simulink model "Energy_Cost03_04_2012"  (Simulink 7.5)
settings: Solver=ode45  StartTime=0.0  StopTime=24  RelTol=1e-3
model workspace: external: MAT-File (data not in the file)
libraries: simulink x4
(part 1 of 2)
settings Model: Creator=jm3gonza  LastModifiedBy=Dr. Juan Miguel Glez
settings DebuggingCC: AlgebraicLoopMsg=none  SolverPrmCheckMsg=none  UnconnectedInputMsg=none  UnconnectedOutputMsg=none  UnconnectedLineMsg=none

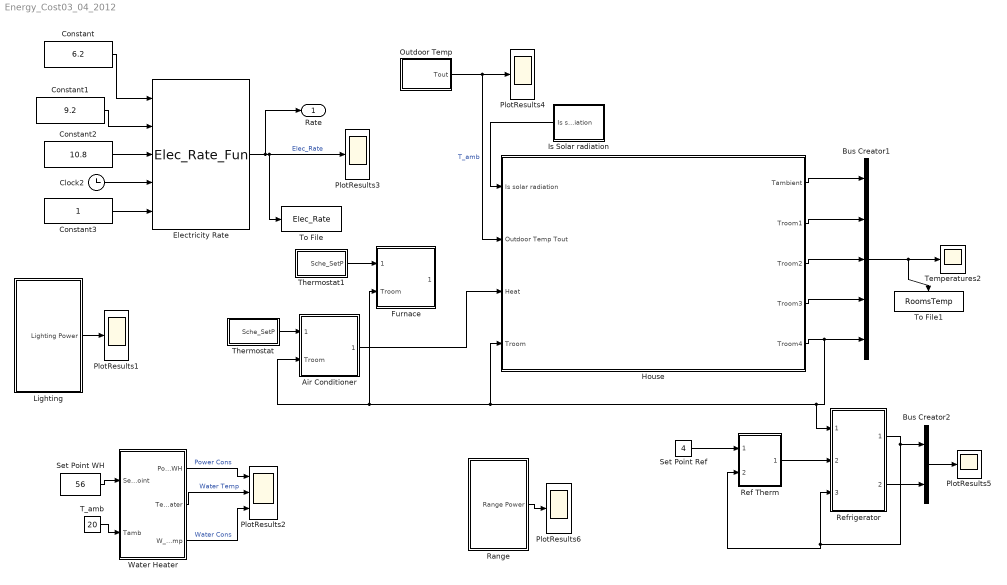
== system Energy_Cost03_04_2012 ==
  Air Conditioner : Subsystem
      mask Display:
      | % plot(-2,-2,10,12,[0 5 5 0 0], [0 0 5 5 0], [5 20 20 5], [0 0 5 5],[0 0 20 20], [5 7 7 5],...
      | %      [5 20], [1 1],[5 20], [2 2],[5 20], [3 3],[5 20], [4 4],...
      | %      [1.5 1.5], [5 7],[3 3], [5 7],[4.5 4.5], [5 7], [6 6], [5 7],[7.5 7.5], [5 7],[9 9], [5 7],...
      | %      [10.5 10.5], [5 7],[12 12], [5 7],[13.5 13.5], [5 7],[15 15], [5 7],[16.5 16.5], [5 7],[17 17], [5 7],[19 19], [5 7],...
      | %      [0 10 30 20], [7 10 10 7], [30 30 20], [10 4 0])
      | image(imread('AA.jpg'))
  Bus Creator1 : BusCreator  Inputs=5
  Bus Creator2 : BusCreator  Inputs=2
  Clock2 : Clock
      settings: Decimation=100
  Constant : Constant  Value=6.2
  Constant1 : Constant  Value=9.2
  Constant2 : Constant  Value=10.8
  Constant3 : Constant
  Electricity Rate : M-S-Function  FunctionName=Elec_Rate_Fun
      mask Display: fprintf('Elec_Rate_Fun %d',[] )
  Furnace : Subsystem
      mask Display:
      | % plot(-2,-2,10,12,[0 5 5 0 0], [0 0 5 5 0], [5 20 20 5], [0 0 5 5],[0 0 20 20], [5 7 7 5],...
      | %      [5 20], [1 1],[5 20], [2 2],[5 20], [3 3],[5 20], [4 4],...
      | %      [1.5 1.5], [5 7],[3 3], [5 7],[4.5 4.5], [5 7], [6 6], [5 7],[7.5 7.5], [5 7],[9 9], [5 7],...
      | %      [10.5 10.5], [5 7],[12 12], [5 7],[13.5 13.5], [5 7],[15 15], [5 7],[16.5 16.5], [5 7],[17 17], [5 7],[19 19], [5 7],...
      | %      [0 10 30 20], [7 10 10 7], [30 30 20], [10 4 0])
      | image(imread('Gas_Furnace.jpg'))
  House : Subsystem
      mask Display:
      | % plot([99.4454661849886;170.309218810871;170.309218810871;99.4454661849886;99.4454661849886], [212.827470386401;212.827470386401;127.790967235342;127.790967235342;212.827470386401])
      | % plot([99.4454661849886;170.309218810871], [184.481969336048;184.481969336048])
      | % plot([133.460067445412;133.460067445412], [184.481969336048;127.790967235342])
      | % plot([241.172971436754;312.036724062636;312.036724062636;241.172971436754;241.172971436754], [212.827470386401;212.827470386401;127.790967235342;127.790967235342;212.827470386401])
      | % plot([241.172971436754;312.036724062636], [184.481969336048;184.481969336048])
      | % plot([275.187572697178;275.187572697178], [184.481969336048;127.790967235342])
      | % plot([113.618216710165;42.7544640842825;368.727726163343;428.253278369084], [453.764229314402;255.34572196193;255.34572196193;453.764229314402])
      | % plot([428.253278369084;499.117030994967], [453.764229314402;382.900476688519])
      | % plot([113.618216710165;428.253278369084], [453.764229314402;453.764229314402])
      | % plot([498.86507098563;499.368991004303], [382.900476688519;382.900476688519])
      | % plot([482.109730364755;496.282480889931], [382.900476688519;382.900476688519])
      | % plot([482.109730364755;374.396826373413], [382.900476688519;275.187572697178])
      | % plot([482.109730364755;425.418728264049], [382.900476688519;439.591478789225])
      | % plot([56.927214609459;56.927214609459;354.554975638166], [255.34572196193;56.927214609459;56.927214609459])
      | % plot([354.554975638166;354.554975638166], [56.927214609459;255.34572196193])
      | % plot([354.554975638166;482.109730364755;482.109730364755], [56.927214609459;184.481969336048;382.900476688519])
      | % plot([397.073227213696;397.073227213696;439.591478789225;439.591478789225;397.073227213696], [170.309218810871;255.34572196193;297.86397353746;209.992920281366;170.309218810871])
      | % plot([397.073227213696;439.591478789225], [227.000220911577;269.518472487107])
      | % plot([419.749628053978;419.749628053978], [246.842071646824;192.985619651154])
      | % patch([0;553.20969549939;553.20969549939;0;0;0.472425017505884;0.47242501750577;552.737270481884;552.737270481885;0.472425017505884;0], [496.518693398684;496.518693398684;0;0;496.518693398684;496.046268381178;0.472425017505884;0.472425017505884;496.046268381178;496.046268381178;496.518693398684], [1;1;1])
      | image(imread('Typical-Canadian-House.jpg'))
  Is Solar radiation : Subsystem
      mask Display:
      | plot([0    0.1500    0.3000    0.4500    1.0000    1.1500    1.3000    1.4500    2.0000    2.1500    2.3000    2.4500    3.0000    3.1500    3.3000    3.4500    4.0000    4.1500    4.3000    4.4500    5.0000    5.1500    5.3000    5.4500    6.0000    6.1500    6.3000    6.4500    7.0000    7.1500    7.3000    7.4500    8.0000    8.1500    8.3000    8.4500    9.0000    9.1500    9.3000    9.4500   10.0000   10.1500   10.3000   10.4500   11.0000   11.1500   11.3000   11.4500   12.0000   12.1500   12.3000   12.4500   13.0000   13.1500   13.3000   13.4500   14.0000   14.1500   14.3000   14.4500   15.0000   15.1500   15.3000   15.4500   16.0000   16.1500   16.3000   16.4500   17.0000   17.1500   17.3000   17.4500   18.0000   18.1500   18.3000   18.4500   19.0000   19.1500   19.3000   19.4500   20.0000   20.1500   20.3000   20.4500   21.0000   21.1500   21.3000   21.4500   22.0000   22.1500   22.3000   22.4500   23.0000   23.1500   23.3000   23.4500],...
      |     [0 0 0 0 0 0 0 0 0 0 0 0 0 0 0 0 0 0 0 0 0 12.85 12.85 12.85 25.699 38.55 51.399 38.55 70.673 70.674 122.073 147.772 102.797 237.697 160.597 186.273 186.268 173.422 404.649 571.658 327.556 411.017 468.811 391.717 314.634 237.577 301.802 417.367 584.316 449.469 719.125 532.917 340.26 199.027 340.266 404.503 288.922 314.601 340.296 301.769 288.938 263.253 288.942 321.049 417.349 327.463 365.947 365.936 269.636 224.709 231.145 173.362 154.103 147.682 128.422 102.737 83.473 70.634 25.685 25.686 0 0 0 0 0 0 0 0 0 0 0 0 0 0 0 0 ])
  Lighting : Subsystem
      mask Display: image(imread('CFL_lighting.jpg'))
  Outdoor Temp : Subsystem
      mask Display:
      | plot([0    0.1500    0.3000    0.4500    1.0000    1.1500    1.3000    1.4500    2.0000    2.1500    2.3000    2.4500    3.0000    3.1500    3.3000    3.4500    4.0000    4.1500    4.3000    4.4500    5.0000    5.1500    5.3000    5.4500    6.0000    6.1500    6.3000    6.4500    7.0000    7.1500    7.3000    7.4500    8.0000    8.1500    8.3000    8.4500    9.0000    9.1500    9.3000    9.4500   10.0000   10.1500   10.3000   10.4500   11.0000   11.1500   11.3000   11.4500   12.0000   12.1500   12.3000   12.4500   13.0000   13.1500   13.3000   13.4500   14.0000   14.1500   14.3000   14.4500   15.0000   15.1500   15.3000   15.4500   16.0000   16.1500   16.3000   16.4500   17.0000   17.1500   17.3000   17.4500   18.0000   18.1500   18.3000   18.4500   19.0000   19.1500   19.3000   19.4500   20.0000   20.1500   20.3000   20.4500   21.0000   21.1500   21.3000   21.4500   22.0000   22.1500   22.3000   22.4500   23.0000   23.1500   23.3000   23.4500],...
      |     [-11.1291  -11.1588  -11.2754  -11.3348  -11.3640  -11.3349  -11.2761  -11.3644  -11.4820  -11.6877  -11.9824  -12.3084  -12.4564  -12.7586 -12.9110  -13.1851  -13.3978  -13.7036  -13.6713  -14.1054  -13.8875  -13.7327  -13.6400  -13.6400  -13.7636  -13.8879  -14.1072  -14.3577  -14.5135  -14.6391  -14.6391  -14.3243  -14.2618  -14.0769  -13.3678  -13.1847  -13.1874  -12.8845  -12.1952  -12.1968  -11.7508  -11.6376  -11.1100  -10.7030  -10.1258   -9.5609   -9.5616   -9.1089   -8.8274   -8.6038   -8.0754   -7.9926   -7.0311   -6.4872   -6.3536   -6.0586   -5.7638   -5.5768   -5.2566   -5.2045   -4.5670   -3.8272   -3.7990   -3.8776   -3.7724   -3.8777   -4.3791   -4.7245   -4.5643   -4.8546   -5.4121  -5.8135   -6.1916   -6.5106   -6.7813   -7.1642   -7.2707   -7.4860   -7.6777   -7.7616   -8.1494   -8.2612   -9.1811   -9.5460  -10.2024  -10.1740  -10.7173  -11.6519  -11.9196  -13.5221  -14.0461  -14.9577  -15.4698  -15.7285  -16.0525  -16.2152])
  PlotResults{1,3..6} (5 alike) : Scope
      PlotResults1 settings: TimeRange=24  YMin=0  YMax=130  SaveName=a1  DataFormat=Array
      PlotResults3 settings: TimeRange=25  YMin=6  YMax=11  SaveName=a  DataFormat=Array
      PlotResults4 settings: TimeRange=24  YMin=-15  YMax=25  SaveName=a3  DataFormat=Array
      PlotResults5 settings: TimeRange=24  YMin=-1  YMax=17  SaveName=a12  DataFormat=Array
      PlotResults6 settings: TimeRange=24  YMin=-1  YMax=1  SaveName=a8  DataFormat=Array
  PlotResults2 : Scope  NumInputPorts=3
      settings: TimeRange=24  YMin=0~51.5~2.5  YMax=4500~58.5~27.5  SaveName=a2  DataFormat=Array
  Range : Subsystem
      mask Display: image(imread('Stove.jpg'))
  Ref Therm : Subsystem
      mask Display: image(imread('Thermostat.jpg'))
  Refrigerator : Subsystem
      mask Display:
      | % plot(-17,-17,180,180,[0 150 150 0 0], [0 0 150 150 0],[0 80 200 150],[150 170 170 150],...
      | %     [150 200 200],[0 30 170],...
      | %     [60 60],[0 150],...
      | %     [50 50 55 55 50],[60 90 90 60 60],...
      | %     [60 60 65 65 60],[60 90 90 60 60])
      | image(imread('Refrigerator.jpg'))
  Set Point Ref : Constant  Value=4
  Set Point WH : Constant  Value=56
  T_amb : Constant  Value=20
  Temperatures2 : Scope
      settings: TimeRange=24  YMin=20  YMax=34  SaveName=a5  DataFormat=Array
  Thermostat : Subsystem
      mask Display: image(imread('Thermostat.jpg'))
  Thermostat1 : Subsystem
      mask Display: image(imread('Thermostat.jpg'))
  To File : ToFile  Filename=Elec_Rate  MatrixName=Elec_Rate
  To File1 : ToFile  Filename=RoomsTemp  MatrixName=RoomsTemp
  Water Heater : Subsystem
      mask Display: image(imread('Water_Heater.jpg'))
  Rate : Outport  InitialOutput=0
  wires:
  Constant/1 -> Electricity Rate/1
  Constant1/1 -> Electricity Rate/2
  Constant2/1 -> Electricity Rate/3
  Clock2/1 -> Electricity Rate/4
  Constant3/1 -> Electricity Rate/5
  Electricity Rate/1 -> PlotResults3/1, To File/1, Rate/1  "Elec_Rate"
  Lighting/1(Lighting Power) -> PlotResults1/1
  Set Point WH/1 -> Water Heater/1(Set point)
  T_amb/1 -> Water Heater/2(Tamb)
  Water Heater/1(Power_WH) -> PlotResults2/1  "Power Cons"
  Water Heater/2(Temp_Water) -> PlotResults2/2  "Water Temp"
  Water Heater/3(W_Consump) -> PlotResults2/3  "Water Cons"
  Outdoor Temp/1(Tout) -> PlotResults4/1, House/2(Outdoor Temp Tout)  "T_amb"
  House/5(Troom4) -> Bus Creator1/5, House/4(Troom), Air Conditioner/2(Troom), Furnace/2(Troom), Refrigerator/1(Outdoor Temp Tout)
  House/1(Tambient) -> Bus Creator1/1
  House/2(Troom1) -> Bus Creator1/2
  House/3(Troom2) -> Bus Creator1/3
  House/4(Troom3) -> Bus Creator1/4
  Bus Creator1/1 -> Temperatures2/1, To File1/1
  Air Conditioner/1(ONOFF) -> House/3(Heat)
  Is Solar radiation/1(Is solar radiation) -> House/1(Is solar radiation)
  Thermostat/1(Sche_SetP) -> Air Conditioner/1(Set point)
  Set Point Ref/1 -> Ref Therm/1(Tamb)
  Bus Creator2/1 -> PlotResults5/1
  Ref Therm/1(Ref Therm) -> Refrigerator/2(On/Off)
  Refrigerator/1(Indoor Temp) -> Bus Creator2/1, Refrigerator/3(Troom), Ref Therm/2(Tamb1)
  Range/1(Range Power) -> PlotResults6/1
  Refrigerator/2(Power_FR) -> Bus Creator2/2
  Thermostat1/1(Sche_SetP) -> Furnace/1(Set point)

== system Energy_Cost03_04_2012/Air Conditioner ==
  Set point : Inport
  Troom : Inport  Port=2
  AA or Heat : Constant
  AA_OnOff : Constant
  Cost_AA : Subsystem
      mask Display: % image(imread('Elec_stove.jpg'))
  PlotResults6 : Scope
      settings: TimeRange=24  YMin=0  YMax=1  SaveName=a9  DataFormat=Array
  Q_AA : Constant  Value=-18991793.6694
  Relay : Relay  OnSwitchValue=1.5  OffSwitchValue=-1.5  OnOutputValue=0  OffOutputValue=1
  Sum : Sum  Inputs=|+-  SampleTime=0  SaturateOnIntegerOverflow=on  InputSameDT=on  OutDataTypeStr=Inherit: Same as first input
  a : Product  Inputs=4  RndMeth=Zero
  ONOFF : Outport  InitialOutput=0
  wires:
  Set point/1 -> Sum/1
  Troom/1 -> Sum/2
  Sum/1 -> Relay/1
  Relay/1 -> a/1, PlotResults6/1
  a/1 -> ONOFF/1, Cost_AA/1(Powe_cons)
  Q_AA/1 -> a/2
  AA_OnOff/1 -> a/3
  AA or Heat/1 -> a/4

== system Energy_Cost03_04_2012/Furnace ==
  Set point : Inport
  Troom : Inport  Port=2
  AA or Heat : Constant
  AA_OnOff : Constant
  Cost_FC : Subsystem
      mask Display: % image(imread('Elec_stove.jpg'))
  PlotResults6 : Scope
      settings: TimeRange=24  YMin=-1  YMax=1  SaveName=a9  DataFormat=Array
  Q_AA : Constant  Value=-42203985.932
  Relay : Relay  OnSwitchValue=1.5  OffSwitchValue=-1.5  OnOutputValue=0  OffOutputValue=1
  Sum : Sum  Inputs=|+-  SampleTime=0  SaturateOnIntegerOverflow=on  InputSameDT=on  OutDataTypeStr=Inherit: Same as first input
  a : Product  Inputs=4  RndMeth=Zero
  ONOFF : Outport  InitialOutput=0
  wires:
  AA or Heat/1 -> a/4
  AA_OnOff/1 -> a/3
  Q_AA/1 -> a/2
  a/1 -> Cost_FC/1(Powe_cons), ONOFF/1
  Relay/1 -> PlotResults6/1, a/1
  Sum/1 -> Relay/1
  Troom/1 -> Sum/2
  Set point/1 -> Sum/1

== system Energy_Cost03_04_2012/House ==
  Is solar radiation : Inport
  Outdoor Temp Tout : Inport  Port=2
  Heat : Inport  Port=3
  Troom : Inport  Port=4
  Room_1 : Subsystem
  Room_2 : Subsystem
  Room_3 : Subsystem
  Room_4 : Subsystem
  Tambient : Outport  InitialOutput=0
  Troom1 : Outport  Port=2  InitialOutput=0
  Troom2 : Outport  Port=3  InitialOutput=0
  Troom3 : Outport  Port=4  InitialOutput=0
  Troom4 : Outport  Port=5  InitialOutput=0
  wires:
  Is solar radiation/1 -> Room_1/1(Is solar radiation), Room_2/1(Is solar radiation), Room_3/1(Is solar radiation), Room_4/1(Is solar radiation)
  Outdoor Temp Tout/1 -> Room_1/2(Outdoor Temp Tout), Room_2/2(Outdoor Temp Tout), Room_3/2(Outdoor Temp Tout), Room_4/2(Outdoor Temp Tout), Tambient/1
  Heat/1 -> Room_1/3(Q_Heat), Room_2/3(Q_Heat), Room_3/3(Q_Heat), Room_4/3(Q_Heat)  "Q_Heat"
  Troom/1 -> Room_1/4(Troom), Room_2/4(Troom), Room_3/4(Troom), Room_4/4(Troom)
  Room_1/1(Room Temp Troom) -> Troom1/1
  Room_2/1(Room Temp Troom) -> Troom2/1
  Room_3/1(Room Temp Troom) -> Troom3/1
  Room_4/1(Room Temp Troom) -> Troom4/1

== system Energy_Cost03_04_2012/Is Solar radiation ==
  Avg Outdoor Temp : Constant
  Outdoor Temp : simulink/Sources/Repeating Sequence Interpolated  SystemSampleTime=-1  OutValues=|  TimeValues=|  LookUpMeth=Interpolation-Use End Values  tsamp=-1  OutMin=[]  OutMax=[]  OutDataTypeStr=double  OutputDataTypeScalingMode=double  OutDataType=fixdt(0,8)  OutScaling=2^-10
      OutValues=|
      | [0
      | 0
      | 0
      | 0
      | 0
      | 0
      | 0
      | 0
      | 0
      | 0
      | 0
      | 0
      | 0
      | 0
      | 0
      | 0
      | 0
      | 0
      | 0
      | 0
      | 0
      | 12.85
      | 12.85
      | 12.85
      | 25.699
      | 38.55
      | 51.399
      | 38.55
      | 70.673
      | 70.674
      | 122.073
      | 147.772
      | 102.797
      | 237.697
      | 160.597
      | 186.273
      | 186.268
      | 173.422
      | 404.649
      | 571.658
      | 327.556
      | 411.017
      | 468.811
      | 391.717
      | 314.634
      | 237.577
      | 301.802
      | 417.367
      | 584.316
      | 449.469
      | 719.125
      | 532.917
      | 340.26
      | 199.027
      | 340.266
      | 404.503
      | 288.922
      | 314.601
      | 340.296
      | 301.769
      | 288.938
      | 263.253
      | 288.942
      | 321.049
      | 417.349
      | 327.463
      | 365.947
      | 365.936
      | 269.636
      | 224.709
      | 231.145
      | 173.362
      | 154.103
      | 147.682
      | 128.422
      | 102.737
      | 83.473
      | 70.634
      | 25.685
      | 25.686
      | 0
      | 0
      | 0
      | 0
      | 0
      | 0
      | 0
      | 0
      | 0
      | 0
      | 0
      | 0
      | 0
      | 0
      | 0
      | 0
      | ].'
      TimeValues=|
      | [         0
      |     0.1500
      |     0.3000
      |     0.4500
      |     1.0000
      |     1.1500
      |     1.3000
      |     1.4500
      |     2.0000
      |     2.1500
      |     2.3000
      |     2.4500
      |     3.0000
      |     3.1500
      |     3.3000
      |     3.4500
      |     4.0000
      |     4.1500
      |     4.3000
      |     4.4500
      |     5.0000
      |     5.1500
      |     5.3000
      |     5.4500
      |     6.0000
      |     6.1500
      |     6.3000
      |     6.4500
      |     7.0000
      |     7.1500
      |     7.3000
      |     7.4500
      |     8.0000
      |     8.1500
      |     8.3000
      |     8.4500
      |     9.0000
      |     9.1500
      |     9.3000
      |     9.4500
      |    10.0000
      |    10.1500
      |    10.3000
      |    10.4500
      |    11.0000
      |    11.1500
      |    11.3000
      |    11.4500
      |    12.0000
      |    12.1500
      |    12.3000
      |    12.4500
      |    13.0000
      |    13.1500
      |    13.3000
      |    13.4500
      |    14.0000
      |    14.1500
      |    14.3000
      |    14.4500
      |    15.0000
      |    15.1500
      |    15.3000
      |    15.4500
      |    16.0000
      |    16.1500
      |    16.3000
      |    16.4500
      |    17.0000
      |    17.1500
      |    17.3000
      |    17.4500
      |    18.0000
      |    18.1500
      |    18.3000
      |    18.4500
      |    19.0000
      |    19.1500
      |    19.3000
      |    19.4500
      |    20.0000
      |    20.1500
      |    20.3000
      |    20.4500
      |    21.0000
      |    21.1500
      |    21.3000
      |    21.4500
      |    22.0000
      |    22.1500
      |    22.3000
      |    22.4500
      |    23.0000
      |    23.1500
      |    23.3000
      |    23.4500].'
  Sum1 : Sum  Inputs=|++  SaturateOnIntegerOverflow=on  InputSameDT=on  OutDataTypeStr=Inherit: Same as first input
  Is solar radiation : Outport  InitialOutput=0
  wires:
  Avg Outdoor Temp/1 -> Sum1/1
  Outdoor Temp/1 -> Sum1/2
  Sum1/1 -> Is solar radiation/1

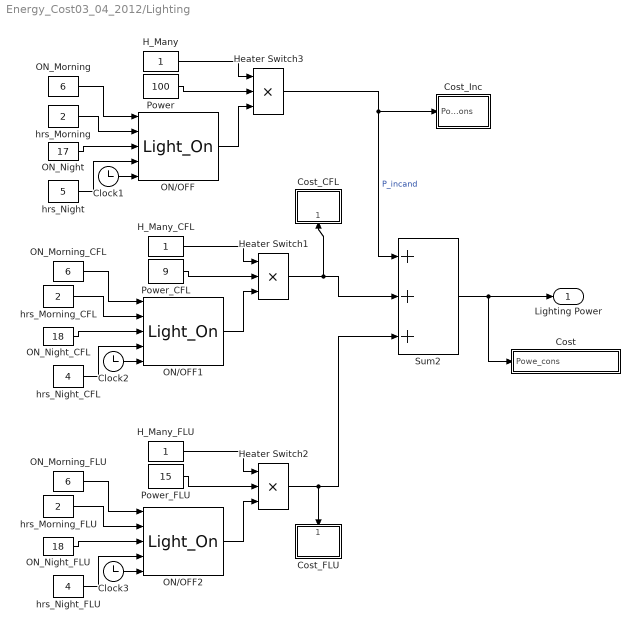
== system Energy_Cost03_04_2012/Lighting ==
  Clock1 : Clock
      settings: Decimation=100
  Clock2 : Clock
      settings: Decimation=100
  Clock3 : Clock
      settings: Decimation=100
  Cost : Subsystem
      mask Display: % image(imread('Elec_stove.jpg'))
  Cost_CFL : Subsystem
      mask Display: % image(imread('Elec_stove.jpg'))
  Cost_FLU : Subsystem
      mask Display: % image(imread('Elec_stove.jpg'))
  Cost_Inc : Subsystem
      mask Display: % image(imread('Elec_stove.jpg'))
  H_Many : Constant
  H_Many_CFL : Constant
  H_Many_FLU : Constant
  Heater Switch1 : Product  Inputs=3  RndMeth=Zero
  Heater Switch2 : Product  Inputs=3  RndMeth=Zero
  Heater Switch3 : Product  Inputs=3  RndMeth=Zero
  ON/OFF : M-S-Function  FunctionName=Light_On
      mask Display: port_label('output', 1, 'ON/OFF')
  ON/OFF1 : M-S-Function  FunctionName=Light_On
      mask Display: port_label('output', 1, 'ON/OFF')
  ON/OFF2 : M-S-Function  FunctionName=Light_On
      mask Display: port_label('output', 1, 'ON/OFF')
  ON_Morning : Constant  Value=6
  ON_Morning_CFL : Constant  Value=6
  ON_Morning_FLU : Constant  Value=6
  ON_Night : Constant  Value=17
  ON_Night_CFL : Constant  Value=18
  ON_Night_FLU : Constant  Value=18
  Power : Constant  Value=100
  Power_CFL : Constant  Value=9
  Power_FLU : Constant  Value=15
  Sum2 : Sum  Inputs=+++  SaturateOnIntegerOverflow=on  InputSameDT=on  OutDataTypeStr=Inherit: Same as first input
  hrs_Morning : Constant  Value=2
  hrs_Morning_CFL : Constant  Value=2
  hrs_Morning_FLU : Constant  Value=2
  hrs_Night : Constant  Value=5
  hrs_Night_CFL : Constant  Value=4
  hrs_Night_FLU : Constant  Value=4
  Lighting Power : Outport  InitialOutput=0
  wires:
  H_Many/1 -> Heater Switch3/1
  Power/1 -> Heater Switch3/2
  Heater Switch3/1 -> Cost_Inc/1(Powe_cons), Sum2/1  "P_incand"
  ON/OFF/1 -> Heater Switch3/3
  Clock1/1 -> ON/OFF/5
  hrs_Morning/1 -> ON/OFF/2
  ON_Night/1 -> ON/OFF/3
  hrs_Night/1 -> ON/OFF/4
  ON_Morning/1 -> ON/OFF/1
  H_Many_CFL/1 -> Heater Switch1/1
  Power_CFL/1 -> Heater Switch1/2
  ON/OFF1/1 -> Heater Switch1/3
  Clock2/1 -> ON/OFF1/5
  hrs_Morning_CFL/1 -> ON/OFF1/2
  ON_Night_CFL/1 -> ON/OFF1/3
  hrs_Night_CFL/1 -> ON/OFF1/4
  ON_Morning_CFL/1 -> ON/OFF1/1
  H_Many_FLU/1 -> Heater Switch2/1
  Power_FLU/1 -> Heater Switch2/2
  ON/OFF2/1 -> Heater Switch2/3
  Clock3/1 -> ON/OFF2/5
  hrs_Morning_FLU/1 -> ON/OFF2/2
  ON_Night_FLU/1 -> ON/OFF2/3
  hrs_Night_FLU/1 -> ON/OFF2/4
  ON_Morning_FLU/1 -> ON/OFF2/1
  Heater Switch1/1 -> Sum2/2, Cost_CFL/1(Powe_cons)
  Heater Switch2/1 -> Sum2/3, Cost_FLU/1(Powe_cons)
  Sum2/1 -> Lighting Power/1, Cost/1(Powe_cons)

== system Energy_Cost03_04_2012/Outdoor Temp ==
  Heater Switch1 : Product  RndMeth=Zero
  Heater Switch2 : Product  RndMeth=Zero
  Sum2 : Sum  SaturateOnIntegerOverflow=on  InputSameDT=on  OutDataTypeStr=Inherit: Same as first input
  Summer : simulink/Sources/Repeating Sequence Interpolated  SystemSampleTime=-1  OutValues=|  TimeValues=|  LookUpMeth=Interpolation-Use End Values  tsamp=-1  OutMin=[]  OutMax=[]  OutDataTypeStr=double  OutputDataTypeScalingMode=double  OutDataType=fixdt(0,8)  OutScaling=2^-10
      OutValues=|
      | [   23.8160
      |    23.7130
      |    23.4480
      |    23.2590
      |    23.1710
      |    23.1330
      |    22.9330
      |    22.8600
      |    22.7100
      |    22.6330
      |    22.4980
      |    22.3130
      |    22.2390
      |    22.1040
      |    21.9830
      |    21.7030
      |    21.5360
      |    21.4650
      |    21.8150
      |    22.1730
      |    22.3830
      |    22.6540
      |    22.7390
      |    22.9630
      |    23.3760
      |    23.9600
      |    24.3460
      |    24.7420
      |    24.9870
      |    25.3280
      |    25.6220
      |    26.4600
      |    26.8940
      |    27.7100
      |    27.9620
      |    28.1630
      |    28.4950
      |    29.0620
      |    29.0190
      |    29.0170
      |    29.2500
      |    29.6940
      |    29.8860
      |    29.9560
      |    30.0730
      |    30.6760
      |    30.8120
      |    30.9150
      |    31.2920
      |    30.8100
      |    31.3250
      |    31.3570
      |    31.6710
      |    32.3710
      |    31.6010
      |    32.0310
      |    32.1090
      |    32.3180
      |    32.3980
      |    31.7870
      |    31.6290
      |    33.0060
      |    33.0040
      |    32.8570
      |    32.9240
      |    32.6620
      |    33.1210
      |    32.6940
      |    32.3640
      |    32.0100
      |    31.5350
      |    32.0310
      |    31.0020
      |    30.4620
      |    30.0880
      |    29.8870
      |    29.5410
      |    29.3690
      |    29.1040
      |    28.6390
      |    28.1200
      |    26.7970
      |    26.0180
      |    25.6170
      |    26.9460
      |    27.3140
      |    27.1220
      |    26.8170
      |    26.5690
      |    26.4040
      |    26.2680
      |    26.1190
      |    25.7690
      |    25.4730
      |    25.2080
      |    24.9570].'
      TimeValues=|
      | [         0
      |     0.1500
      |     0.3000
      |     0.4500
      |     1.0000
      |     1.1500
      |     1.3000
      |     1.4500
      |     2.0000
      |     2.1500
      |     2.3000
      |     2.4500
      |     3.0000
      |     3.1500
      |     3.3000
      |     3.4500
      |     4.0000
      |     4.1500
      |     4.3000
      |     4.4500
      |     5.0000
      |     5.1500
      |     5.3000
      |     5.4500
      |     6.0000
      |     6.1500
      |     6.3000
      |     6.4500
      |     7.0000
      |     7.1500
      |     7.3000
      |     7.4500
      |     8.0000
      |     8.1500
      |     8.3000
      |     8.4500
      |     9.0000
      |     9.1500
      |     9.3000
      |     9.4500
      |    10.0000
      |    10.1500
      |    10.3000
      |    10.4500
      |    11.0000
      |    11.1500
      |    11.3000
      |    11.4500
      |    12.0000
      |    12.1500
      |    12.3000
      |    12.4500
      |    13.0000
      |    13.1500
      |    13.3000
      |    13.4500
      |    14.0000
      |    14.1500
      |    14.3000
      |    14.4500
      |    15.0000
      |    15.1500
      |    15.3000
      |    15.4500
      |    16.0000
      |    16.1500
      |    16.3000
      |    16.4500
      |    17.0000
      |    17.1500
      |    17.3000
      |    17.4500
      |    18.0000
      |    18.1500
      |    18.3000
      |    18.4500
      |    19.0000
      |    19.1500
      |    19.3000
      |    19.4500
      |    20.0000
      |    20.1500
      |    20.3000
      |    20.4500
      |    21.0000
      |    21.1500
      |    21.3000
      |    21.4500
      |    22.0000
      |    22.1500
      |    22.3000
      |    22.4500
      |    23.0000
      |    23.1500
      |    23.3000
      |    23.4500].'
  Temp_aux : Constant  SampleTime=0
  Temp_aux1 : Constant  Value=0  SampleTime=0
  Winter : simulink/Sources/Repeating Sequence Interpolated  SystemSampleTime=-1  OutValues=|  TimeValues=|  LookUpMeth=Interpolation-Use End Values  tsamp=-1  OutMin=[]  OutMax=[]  OutDataTypeStr=double  OutputDataTypeScalingMode=double  OutDataType=fixdt(0,8)  OutScaling=2^-10
      OutValues=|
      | [  -11.1291
      |   -11.1588
      |   -11.2754
      |   -11.3348
      |   -11.3640
      |   -11.3349
      |   -11.2761
      |   -11.3644
      |   -11.4820
      |   -11.6877
      |   -11.9824
      |   -12.3084
      |   -12.4564
      |   -12.7586
      |   -12.9110
      |   -13.1851
      |   -13.3978
      |   -13.7036
      |   -13.6713
      |   -14.1054
      |   -13.8875
      |   -13.7327
      |   -13.6400
      |   -13.6400
      |   -13.7636
      |   -13.8879
      |   -14.1072
      |   -14.3577
      |   -14.5135
      |   -14.6391
      |   -14.6391
      |   -14.3243
      |   -14.2618
      |   -14.0769
      |   -13.3678
      |   -13.1847
      |   -13.1874
      |   -12.8845
      |   -12.1952
      |   -12.1968
      |   -11.7508
      |   -11.6376
      |   -11.1100
      |   -10.7030
      |   -10.1258
      |    -9.5609
      |    -9.5616
      |    -9.1089
      |    -8.8274
      |    -8.6038
      |    -8.0754
      |    -7.9926
      |    -7.0311
      |    -6.4872
      |    -6.3536
      |    -6.0586
      |    -5.7638
      |    -5.5768
      |    -5.2566
      |    -5.2045
      |    -4.5670
      |    -3.8272
      |    -3.7990
      |    -3.8776
      |    -3.7724
      |    -3.8777
      |    -4.3791
      |    -4.7245
      |    -4.5643
      |    -4.8546
      |    -5.4121
      |    -5.8135
      |    -6.1916
      |    -6.5106
      |    -6.7813
      |    -7.1642
      |    -7.2707
      |    -7.4860
      |    -7.6777
      |    -7.7616
      |    -8.1494
      |    -8.2612
      |    -9.1811
      |    -9.5460
      |   -10.2024
      |   -10.1740
      |   -10.7173
      |   -11.6519
      |   -11.9196
      |   -13.5221
      |   -14.0461
      |   -14.9577
      |   -15.4698
      |   -15.7285
      |   -16.0525
      |   -16.2152
      |   -16.2152
      |   -16.52].'
      TimeValues=|
      | [         0
      |     0.1500
      |     0.3000
      |     0.4500
      |     1.0000
      |     1.1500
      |     1.3000
      |     1.4500
      |     2.0000
      |     2.1500
      |     2.3000
      |     2.4500
      |     3.0000
      |     3.1500
      |     3.3000
      |     3.4500
      |     4.0000
      |     4.1500
      |     4.3000
      |     4.4500
      |     5.0000
      |     5.1500
      |     5.3000
      |     5.4500
      |     6.0000
      |     6.1500
      |     6.3000
      |     6.4500
      |     7.0000
      |     7.1500
      |     7.3000
      |     7.4500
      |     8.0000
      |     8.1500
      |     8.3000
      |     8.4500
      |     9.0000
      |     9.1500
      |     9.3000
      |     9.4500
      |    10.0000
      |    10.1500
      |    10.3000
      |    10.4500
      |    11.0000
      |    11.1500
      |    11.3000
      |    11.4500
      |    12.0000
      |    12.1500
      |    12.3000
      |    12.4500
      |    13.0000
      |    13.1500
      |    13.3000
      |    13.4500
      |    14.0000
      |    14.1500
      |    14.3000
      |    14.4500
      |    15.0000
      |    15.1500
      |    15.3000
      |    15.4500
      |    16.0000
      |    16.1500
      |    16.3000
      |    16.4500
      |    17.0000
      |    17.1500
      |    17.3000
      |    17.4500
      |    18.0000
      |    18.1500
      |    18.3000
      |    18.4500
      |    19.0000
      |    19.1500
      |    19.3000
      |    19.4500
      |    20.0000
      |    20.1500
      |    20.3000
      |    20.4500
      |    21.0000
      |    21.1500
      |    21.3000
      |    21.4500
      |    22.0000
      |    22.1500
      |    22.3000
      |    22.4500
      |    23.0000
      |    23.1500
      |    23.3000
      |    23.4500
      |    23.900  
      |    24.000].'
  Tout : Outport  InitialOutput=0
  wires:
  Heater Switch1/1 -> Sum2/1  "Toutdoors"
  Temp_aux/1 -> Heater Switch1/1
  Summer/1 -> Heater Switch1/2
  Heater Switch2/1 -> Sum2/2  "Toutdoors"
  Temp_aux1/1 -> Heater Switch2/1
  Winter/1 -> Heater Switch2/2
  Sum2/1 -> Tout/1

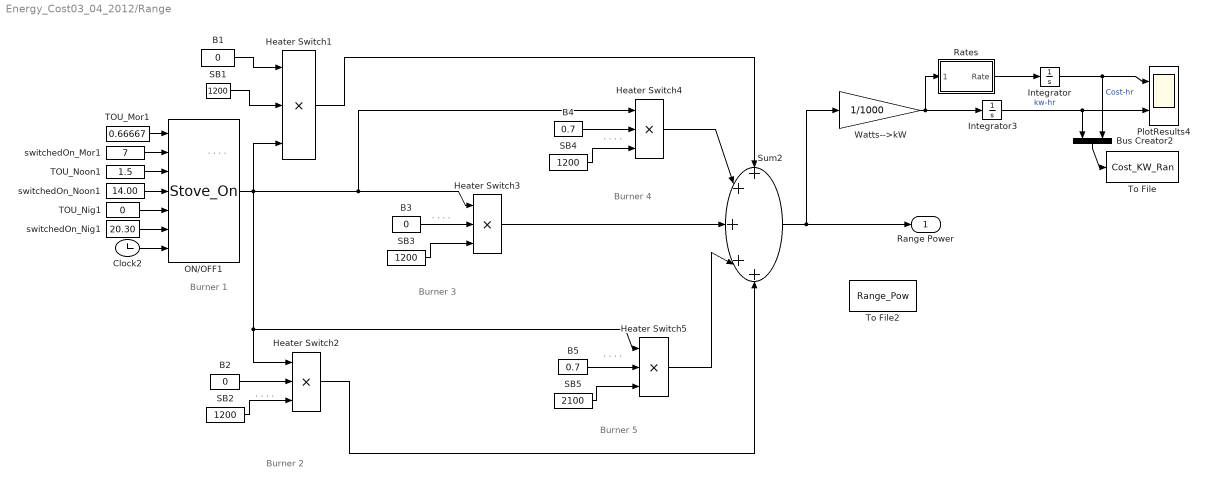
== system Energy_Cost03_04_2012/Range ==
  note: Burner 1
  note: Burner 2
  note: Burner 3
  note: Burner 4
  note: Burner 5
  note: .                                                                                     .
      |
      |
      |
      |
      |
      |
      |
      |
      |
      |
      |
      |
      |
      |
      |
      |
      |
      |
      | .                                                                                     .
  note: .                                             .
      |
      |
      |
      |
      |
      |
      | .                                             .
  note: .                                             .
      |
      |
      |
      |
      |
      |
      | .                                             .
  note: .                                             .
      |
      |
      |
      |
      |
      |
      | .                                             .
  note: .                                             .
      |
      |
      |
      |
      |
      |
      | .                                             .
  B1 : Constant  Value=0
  B2 : Constant  Value=0
  B3 : Constant  Value=0
  B4 : Constant  Value=0.7
  B5 : Constant  Value=0.7
  Bus Creator2 : BusCreator  Inputs=2
  Clock2 : Clock
      settings: Decimation=100
  Heater Switch{1..5} (5 alike) : Product  Inputs=3  RndMeth=Zero
  Integrator : Integrator
  Integrator3 : Integrator
  ON/OFF1 : M-S-Function  FunctionName=Stove_On
      mask Display: port_label('output', 1, 'ON/OFF')
  PlotResults4 : Scope  NumInputPorts=2
      settings: TimeRange=24  YMin=0~0  YMax=37.5~3.75  SaveName=a17  DataFormat=Array
  Rates : Subsystem
      mask Display: % image(imread('Elec_stove.jpg'))
  SB{1..4} (4 alike) : Constant  Value=1200
  SB5 : Constant  Value=2100
  Sum2 : Sum  Inputs=+++++  SaturateOnIntegerOverflow=on  InputSameDT=on  OutDataTypeStr=Inherit: Same as first input
  TOU_Mor1 : Constant  Value=0.66667
  TOU_Nig1 : Constant  Value=0
  TOU_Noon1 : Constant  Value=1.5
  To File : ToFile  Filename=Cost_KW_Ran  MatrixName=Cost_KW
  To File2 : ToFile  Filename=Range_Pow  MatrixName=Range_Pow
  Watts-->kW : Gain  Gain=1/1000  SaturateOnIntegerOverflow=on  OutDataTypeStr=Inherit: Same as input  ParamDataTypeStr=Inherit: Same as input
  switchedOn_Mor1 : Constant  Value=7
  switchedOn_Nig1 : Constant  Value=20.30
  switchedOn_Noon1 : Constant  Value=14.00
  Range Power : Outport  InitialOutput=0
  wires:
  Rates/1(Rate) -> Integrator/1
  Watts-->kW/1 -> Integrator3/1, Rates/1(Powe_cons)
  Integrator3/1 -> PlotResults4/2, Bus Creator2/1  "kw-hr"
  Bus Creator2/1 -> To File/1
  Integrator/1 -> PlotResults4/1, Bus Creator2/2  "Cost-hr"
  TOU_Mor1/1 -> ON/OFF1/1
  switchedOn_Mor1/1 -> ON/OFF1/2
  Clock2/1 -> ON/OFF1/7
  TOU_Noon1/1 -> ON/OFF1/3
  switchedOn_Noon1/1 -> ON/OFF1/4
  TOU_Nig1/1 -> ON/OFF1/5
  switchedOn_Nig1/1 -> ON/OFF1/6
  B1/1 -> Heater Switch1/1
  SB1/1 -> Heater Switch1/2
  ON/OFF1/1 -> Heater Switch1/3, Heater Switch3/1, Heater Switch4/1, Heater Switch2/1, Heater Switch5/1
  SB2/1 -> Heater Switch2/3
  B2/1 -> Heater Switch2/2
  SB3/1 -> Heater Switch3/3
  B3/1 -> Heater Switch3/2
  SB4/1 -> Heater Switch4/3
  B4/1 -> Heater Switch4/2
  SB5/1 -> Heater Switch5/3
  B5/1 -> Heater Switch5/2
  Heater Switch1/1 -> Sum2/1
  Heater Switch4/1 -> Sum2/2
  Heater Switch3/1 -> Sum2/3
  Heater Switch5/1 -> Sum2/4
  Heater Switch2/1 -> Sum2/5
  Sum2/1 -> Range Power/1, Watts-->kW/1

== system Energy_Cost03_04_2012/Ref Therm ==
  Tamb : Inport
  Tamb1 : Inport  Port=2
  Sum3 : Sum  Inputs=|+-  SampleTime=0  SaturateOnIntegerOverflow=on  InputSameDT=on  OutDataTypeStr=Inherit: Same as first input
  Thermostat1 : Relay  OnSwitchValue=1.5  OffSwitchValue=-1.5  OnOutputValue=0  OffOutputValue=1  ZeroCross=off  SampleTime=0.14
  Ref Therm : Outport  InitialOutput=0
  wires:
  Sum3/1 -> Thermostat1/1
  Thermostat1/1 -> Ref Therm/1
  Tamb/1 -> Sum3/1
  Tamb1/1 -> Sum3/2

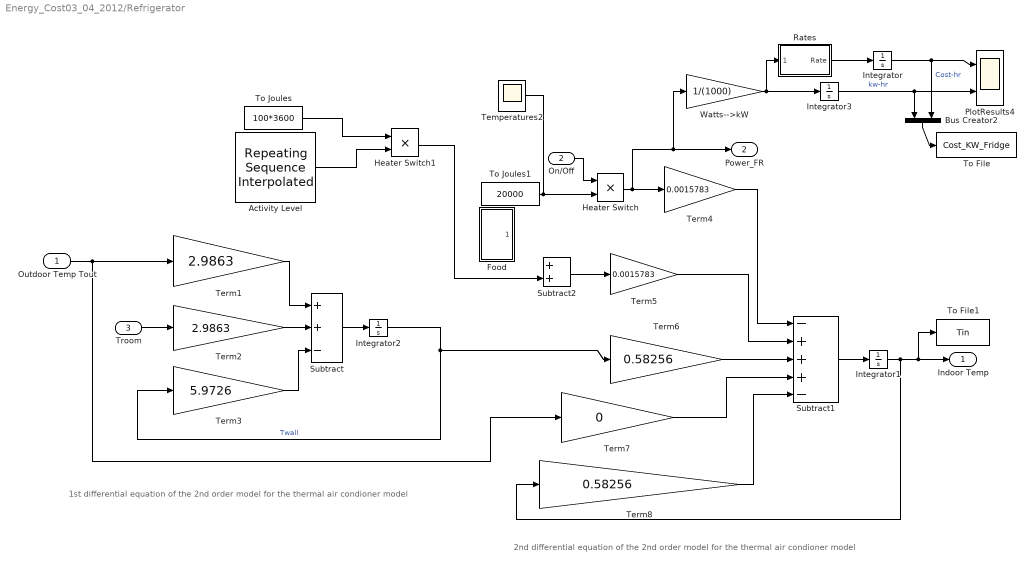
== system Energy_Cost03_04_2012/Refrigerator ==
  note: 1st differential equation of the 2nd order
      | model for the thermal air condioner model
  note: 2nd differential equation of the 2nd order
      | model for the thermal air condioner model
  Outdoor Temp Tout : Inport
  On/Off : Inport  Port=2
  Troom : Inport  Port=3
  Activity Level : simulink/Sources/Repeating Sequence Interpolated  SystemSampleTime=-1  OutValues=|  TimeValues=|  LookUpMeth=Interpolation-Use End Values  tsamp=0.1  OutMin=[]  OutMax=[]  OutDataTypeStr=double  OutputDataTypeScalingMode=double  OutDataType=fixdt(0,8)  OutScaling=2^-10
      OutValues=|
      | [         0
      |          0
      |     0.0700
      |     0.0700
      |          0
      |          0
      |     0.1000
      |     0.1000
      |          0
      |          0
      |     0.1300
      |     0.1300
      |          0
      |          0
      |     0.0300
      |     0.0300
      |          0
      |          0
      |          0
      |     0.0700
      |     0.0700
      |          0
      |          0
      |     0.1700
      |     0.1700
      |          0
      |          0
      |     0.2300
      |     0.2300
      |          0
      |          0
      |     0.1300
      |     0.1300
      |          0
      |          0
      |     0.0700
      |     0.0700
      |          0
      |          0].'
      TimeValues=|
      | [                   0
      |    9.299899999999999
      |    9.300000000000001
      |    9.303990000000001
      |    9.304000000000000
      |    9.749000000000001
      |    9.750000000000000
      |    9.755000000000001
      |    9.756000000000000
      |    9.999000000000001
      |   10.000000000000000
      |   10.006700000000000
      |   10.006800000000000
      |   10.149900000000001
      |   10.150000000000000
      |   10.151600000000000
      |   10.151700000000000
      |   10.300100000000000
      |   13.299899999999999
      |   13.300000000000001
      |   13.303300000000000
      |   13.303400000000000
      |   13.449900000000000
      |   13.449999999999999
      |   13.458399999999999
      |   13.458500000000001
      |   13.999900000000000
      |   14.000000000000000
      |   14.011690000000000
      |   14.011699999999999
      |   14.149900000000001
      |   14.150000000000000
      |   14.156700000000001
      |   14.156800000000000
      |   14.299899999999999
      |   14.300000000000001
      |   14.303300000000000
      |   14.303400000000000
      |   24.000000000000000].'
  Bus Creator2 : BusCreator  Inputs=2
  Food : Subsystem
  Heater Switch : Product  RndMeth=Zero
  Heater Switch1 : Product  RndMeth=Zero
  Integrator : Integrator
  Integrator1 : Integrator  InitialCondition=4
  Integrator2 : Integrator  InitialCondition=21
  Integrator3 : Integrator
  PlotResults4 : Scope  NumInputPorts=2
      settings: TimeRange=24  YMin=32.5~5.5  YMax=70~11.25  SaveName=a7  DataFormat=Array
  Rates : Subsystem
      mask Display: % image(imread('Elec_stove.jpg'))
  Subtract : Sum  Inputs=++-
  Subtract1 : Sum  Inputs=-+++-
  Subtract2 : Sum
  Temperatures2 : Scope
      settings: TimeRange=24  YMin=0  YMax=21000  SaveName=a13  DataFormat=Array
  Term1 : Gain  Gain=2.9863
  Term2 : Gain  Gain=2.9863
  Term3 : Gain  Gain=5.9726
  Term4 : Gain  Gain=0.0015783
  Term5 : Gain  Gain=0.0015783
  Term6 : Gain  Gain=0.58256
  Term7 : Gain  Gain=0
  Term8 : Gain  Gain=0.58256
  To File : ToFile  Filename=Cost_KW_Fridge  MatrixName=Cost_KW_Fridge
  To File1 : ToFile  Filename=Tin  MatrixName=Tin
  To Joules : Constant  Value=100*3600
  To Joules1 : Constant  Value=20000
  Watts-->kW : Gain  Gain=1/(1000)  SaturateOnIntegerOverflow=on  OutDataTypeStr=Inherit: Same as input  ParamDataTypeStr=Inherit: Same as input
  Indoor Temp : Outport  InitialOutput=0
  Power_FR : Outport  Port=2  InitialOutput=0
  wires:
  Term3/1 -> Subtract/3
  Subtract/1 -> Integrator2/1
  Integrator2/1 -> Term3/1, Term6/1  "Twall"
  Integrator1/1 -> Indoor Temp/1, To File1/1, Term8/1
  Subtract1/1 -> Integrator1/1
  Outdoor Temp Tout/1 -> Term7/1, Term1/1
  Troom/1 -> Term2/1
  Term5/1 -> Subtract1/2
  Term6/1 -> Subtract1/3
  Term7/1 -> Subtract1/4
  Term8/1 -> Subtract1/5
  Activity Level/1 -> Heater Switch1/2
  To Joules/1 -> Heater Switch1/1
  Heater Switch1/1 -> Subtract2/2
  On/Off/1 -> Heater Switch/1
  Subtract2/1 -> Term5/1
  Term1/1 -> Subtract/1
  Term2/1 -> Subtract/2
  To Joules1/1 -> Temperatures2/1, Heater Switch/2
  Heater Switch/1 -> Term4/1, Power_FR/1, Watts-->kW/1
  Term4/1 -> Subtract1/1
  Rates/1(Rate) -> Integrator/1
  Watts-->kW/1 -> Integrator3/1, Rates/1(Powe_cons)
  Integrator3/1 -> PlotResults4/2, Bus Creator2/1  "kw-hr"
  Bus Creator2/1 -> To File/1
  Integrator/1 -> PlotResults4/1, Bus Creator2/2  "Cost-hr"

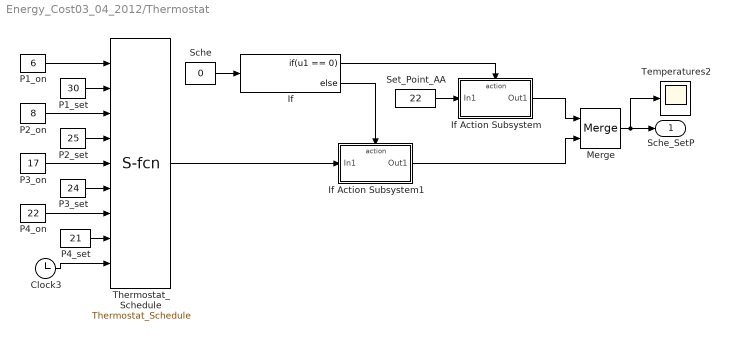
== system Energy_Cost03_04_2012/Thermostat ==
  Clock3 : Clock
      settings: Decimation=100
  If : If  IfExpression=u1 == 0
  If Action Subsystem : Subsystem  TreatAsAtomicUnit=on
  If Action Subsystem1 : Subsystem  TreatAsAtomicUnit=on
  Merge : Merge
  P1_on : Constant  Value=6
  P1_set : Constant  Value=30
  P2_on : Constant  Value=8
  P2_set : Constant  Value=25
  P3_on : Constant  Value=17
  P3_set : Constant  Value=24
  P4_on : Constant  Value=22
  P4_set : Constant  Value=21
  Sche : Constant  Value=0
  Set_Point_AA : Constant  Value=22
  Temperatures2 : Scope
      settings: TimeRange=24  YMin=21  YMax=21  SaveName=a4  DataFormat=Array
  Thermostat_Schedule : M-S-Function  FunctionName=Thermostat_Schedule
      mask Display: port_label('output', 1, 'ON/OFF')
  Sche_SetP : Outport  InitialOutput=0
  wires:
  P1_on/1 -> Thermostat_Schedule/1
  P1_set/1 -> Thermostat_Schedule/2
  P2_on/1 -> Thermostat_Schedule/3
  P2_set/1 -> Thermostat_Schedule/4
  P3_on/1 -> Thermostat_Schedule/5
  P3_set/1 -> Thermostat_Schedule/6
  P4_on/1 -> Thermostat_Schedule/7
  P4_set/1 -> Thermostat_Schedule/8
  Clock3/1 -> Thermostat_Schedule/9
  Sche/1 -> If/1
  If/1 -> If Action Subsystem/Action
  Set_Point_AA/1 -> If Action Subsystem/1(In1)
  If/2 -> If Action Subsystem1/Action
  Merge/1 -> Sche_SetP/1, Temperatures2/1
  Thermostat_Schedule/1 -> If Action Subsystem1/1(In1)
  If Action Subsystem1/1(Out1) -> Merge/2
  If Action Subsystem/1(Out1) -> Merge/1

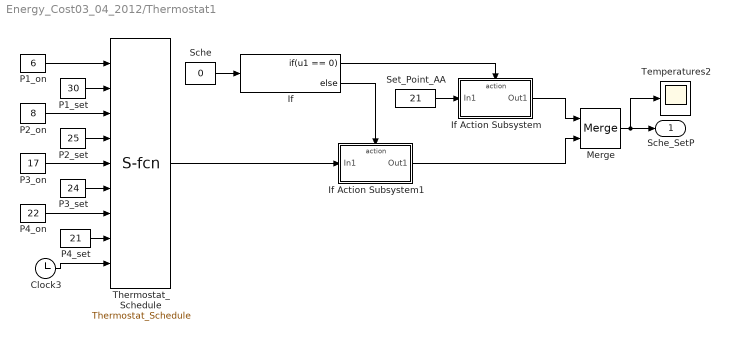
== system Energy_Cost03_04_2012/Thermostat1 ==
  Clock3 : Clock
      settings: Decimation=100
  If : If  IfExpression=u1 == 0
  If Action Subsystem : Subsystem  TreatAsAtomicUnit=on
  If Action Subsystem1 : Subsystem  TreatAsAtomicUnit=on
  Merge : Merge
  P1_on : Constant  Value=6
  P1_set : Constant  Value=30
  P2_on : Constant  Value=8
  P2_set : Constant  Value=25
  P3_on : Constant  Value=17
  P3_set : Constant  Value=24
  P4_on : Constant  Value=22
  P4_set : Constant  Value=21
  Sche : Constant  Value=0
  Set_Point_AA : Constant  Value=21
  Temperatures2 : Scope
      settings: TimeRange=24  YMin=21  YMax=21  SaveName=a4  DataFormat=Array
  Thermostat_Schedule : M-S-Function  FunctionName=Thermostat_Schedule
      mask Display: port_label('output', 1, 'ON/OFF')
  Sche_SetP : Outport  InitialOutput=0
  wires:
  P1_on/1 -> Thermostat_Schedule/1
  P1_set/1 -> Thermostat_Schedule/2
  P2_on/1 -> Thermostat_Schedule/3
  P2_set/1 -> Thermostat_Schedule/4
  P3_on/1 -> Thermostat_Schedule/5
  P3_set/1 -> Thermostat_Schedule/6
  P4_on/1 -> Thermostat_Schedule/7
  P4_set/1 -> Thermostat_Schedule/8
  Clock3/1 -> Thermostat_Schedule/9
  Sche/1 -> If/1
  If/1 -> If Action Subsystem/Action
  Set_Point_AA/1 -> If Action Subsystem/1(In1)
  If/2 -> If Action Subsystem1/Action
  Merge/1 -> Sche_SetP/1, Temperatures2/1
  Thermostat_Schedule/1 -> If Action Subsystem1/1(In1)
  If Action Subsystem1/1(Out1) -> Merge/2
  If Action Subsystem/1(Out1) -> Merge/1

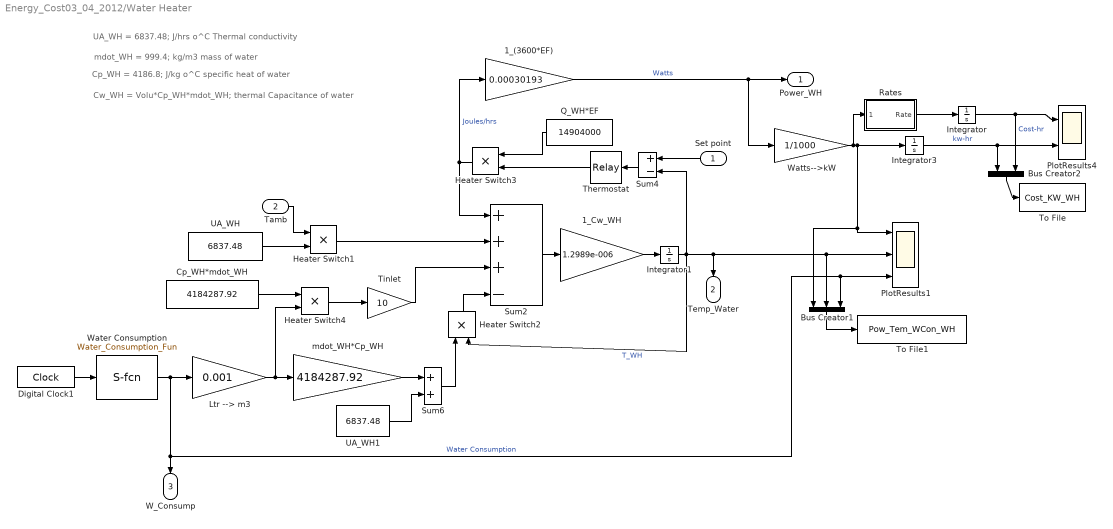
== system Energy_Cost03_04_2012/Water Heater ==
  note: UA_WH = 6837.48; J/hrs o^C Thermal conductivity
  note: mdot_WH = 999.4; kg/m3 mass of water
  note: Cp_WH = 4186.8; J/kg o^C specific heat of water
  note: Cw_WH = Volu*Cp_WH*mdot_WH; thermal Capacitance of water
  Set point : Inport
  Tamb : Inport  Port=2
  1_(3600*EF) : Gain  Gain=0.00030193  SaturateOnIntegerOverflow=on  OutDataTypeStr=Inherit: Same as input  ParamDataTypeStr=Inherit: Same as input
  1_Cw_WH : Gain  Gain=1.2989e-006  SaturateOnIntegerOverflow=on  OutDataTypeStr=Inherit: Same as input  ParamDataTypeStr=Inherit: Same as input
  Bus Creator1 : BusCreator  Inputs=3
  Bus Creator2 : BusCreator  Inputs=2
  Cp_WH*mdot_WH : Constant  Value=4184287.92
  Digital Clock1 : DigitalClock
  Heater Switch{1..4} (4 alike) : Product  RndMeth=Zero
  Integrator : Integrator
  Integrator1 : Integrator  InitialCondition=55
  Integrator3 : Integrator
  Ltr --> m3 : Gain  Gain=0.001
  PlotResults1 : Scope  NumInputPorts=3
      settings: TimeRange=24  YMin=0~42~2.5  YMax=4.5~55~27.5  SaveName=a11  DataFormat=Array
  PlotResults4 : Scope  NumInputPorts=2
      settings: TimeRange=24  YMin=47.5~13.75  YMax=67.5~18.5  SaveName=a14  DataFormat=Array
  Q_WH*EF : Constant  Value=14904000  VectorParams1D=off
  Rates : Subsystem
      mask Display: % image(imread('Elec_stove.jpg'))
  Sum2 : Sum  Inputs=+++-  SaturateOnIntegerOverflow=on  InputSameDT=on  OutDataTypeStr=Inherit: Same as first input
  Sum4 : Sum  Inputs=+-  SaturateOnIntegerOverflow=on  InputSameDT=on  OutDataTypeStr=Inherit: Same as first input
  Sum6 : Sum  SaturateOnIntegerOverflow=on  InputSameDT=on  OutDataTypeStr=Inherit: Same as first input
  Thermostat : Relay  OnSwitchValue=3  OffSwitchValue=-3
  Tinlet : Gain  Gain=10  SaturateOnIntegerOverflow=on  OutDataTypeStr=Inherit: Same as input  ParamDataTypeStr=Inherit: Same as input
  To File : ToFile  Filename=Cost_KW_WH  MatrixName=Cost_KW_WH
  To File1 : ToFile  Filename=Pow_Tem_WCon_WH  MatrixName=Pow_Tem_WCon_WH
  UA_WH : Constant  Value=6837.48
  UA_WH1 : Constant  Value=6837.48
  Water Consumption : M-S-Function  FunctionName=Water_Consumption_Fun
      mask Display: image(imread('Water_Cons.jpg'))
  Watts-->kW : Gain  Gain=1/1000  SaturateOnIntegerOverflow=on  OutDataTypeStr=Inherit: Same as input  ParamDataTypeStr=Inherit: Same as input
  mdot_WH*Cp_WH : Gain  Gain=4184287.92  SaturateOnIntegerOverflow=on  OutDataTypeStr=Inherit: Same as input  ParamDataTypeStr=Inherit: Same as input
  Power_WH : Outport  InitialOutput=0
  Temp_Water : Outport  Port=2  InitialOutput=0
  W_Consump : Outport  Port=3  InitialOutput=0
  wires:
  Sum2/1 -> 1_Cw_WH/1
  1_Cw_WH/1 -> Integrator1/1
  Digital Clock1/1 -> Water Consumption/1
  Water Consumption/1 -> Ltr --> m3/1, W_Consump/1, PlotResults1/3, Bus Creator1/3  "Water Consumption"
  UA_WH/1 -> Heater Switch1/2
  Ltr --> m3/1 -> mdot_WH*Cp_WH/1, Heater Switch4/2
  mdot_WH*Cp_WH/1 -> Sum6/1
  UA_WH1/1 -> Sum6/2
  Sum6/1 -> Heater Switch2/1
  Integrator1/1 -> Heater Switch2/2, Sum4/2, Temp_Water/1, PlotResults1/2, Bus Creator1/2  "T_WH"
  Heater Switch2/1 -> Sum2/4
  Cp_WH*mdot_WH/1 -> Heater Switch4/1
  Heater Switch4/1 -> Tinlet/1
  Tinlet/1 -> Sum2/3
  Heater Switch1/1 -> Sum2/2
  Set point/1 -> Sum4/1
  Sum4/1 -> Thermostat/1
  Q_WH*EF/1 -> Heater Switch3/1
  Heater Switch3/1 -> Sum2/1, 1_(3600*EF)/1  "Joules/hrs"
  1_(3600*EF)/1 -> Power_WH/1, Watts-->kW/1  "Watts"
  Thermostat/1 -> Heater Switch3/2
  Tamb/1 -> Heater Switch1/1
  Rates/1(Rate) -> Integrator/1
  Watts-->kW/1 -> Rates/1(Powe_cons), Integrator3/1, PlotResults1/1, Bus Creator1/1
  Integrator3/1 -> PlotResults4/2, Bus Creator2/1  "kw-hr"
  Bus Creator2/1 -> To File/1
  Bus Creator1/1 -> To File1/1
  Integrator/1 -> PlotResults4/1, Bus Creator2/2  "Cost-hr"

== system Energy_Cost03_04_2012/Air Conditioner/Cost_AA ==
  Powe_cons : Inport
  Bus Creator2 : BusCreator  Inputs=3
  Integrator : Integrator
  Integrator3 : Integrator
  PlotResults4 : Scope  NumInputPorts=2
      settings: TimeRange=24  YMin=675~70.5  YMax=705~75  SaveName=a18  DataFormat=Array
  Rates : Subsystem
      mask Display: % image(imread('Elec_stove.jpg'))
  To File : ToFile  Filename=Pow_Cost_AC  MatrixName=Pow_Cost_AC
  Watts-->kW : Gain  Gain=-1/(3600*1000)  SaturateOnIntegerOverflow=on  OutDataTypeStr=Inherit: Same as input  ParamDataTypeStr=Inherit: Same as input
  wires:
  Rates/1(Rate) -> Integrator/1
  Watts-->kW/1 -> Rates/1(Powe_cons), Integrator3/1, Bus Creator2/1
  Integrator3/1 -> PlotResults4/2, Bus Creator2/2  "kw_hr"
  Bus Creator2/1 -> To File/1
  Integrator/1 -> PlotResults4/1, Bus Creator2/3  "Cost_hr"
  Powe_cons/1 -> Watts-->kW/1

== system Energy_Cost03_04_2012/Furnace/Cost_FC ==
  Powe_cons : Inport
  Bus Creator2 : BusCreator  Inputs=3
  Integrator : Integrator
  Integrator3 : Integrator
  PlotResults4 : Scope  NumInputPorts=2
      settings: TimeRange=24  YMin=925~98  YMax=1035~108.5  SaveName=a18  DataFormat=Array
  Rates : Subsystem
      mask Display: % image(imread('Elec_stove.jpg'))
  To File : ToFile  Filename=Cost_FC  MatrixName=Cost_FC
  Watts-->kW : Gain  Gain=-1/(3600*1000)  SaturateOnIntegerOverflow=on  OutDataTypeStr=Inherit: Same as input  ParamDataTypeStr=Inherit: Same as input
  wires:
  Powe_cons/1 -> Watts-->kW/1
  Integrator/1 -> Bus Creator2/3, PlotResults4/1  "Cost_hr"
  Bus Creator2/1 -> To File/1
  Integrator3/1 -> Bus Creator2/2, PlotResults4/2  "kw_hr"
  Watts-->kW/1 -> Bus Creator2/1, Integrator3/1, Rates/1(Powe_cons)
  Rates/1(Rate) -> Integrator/1

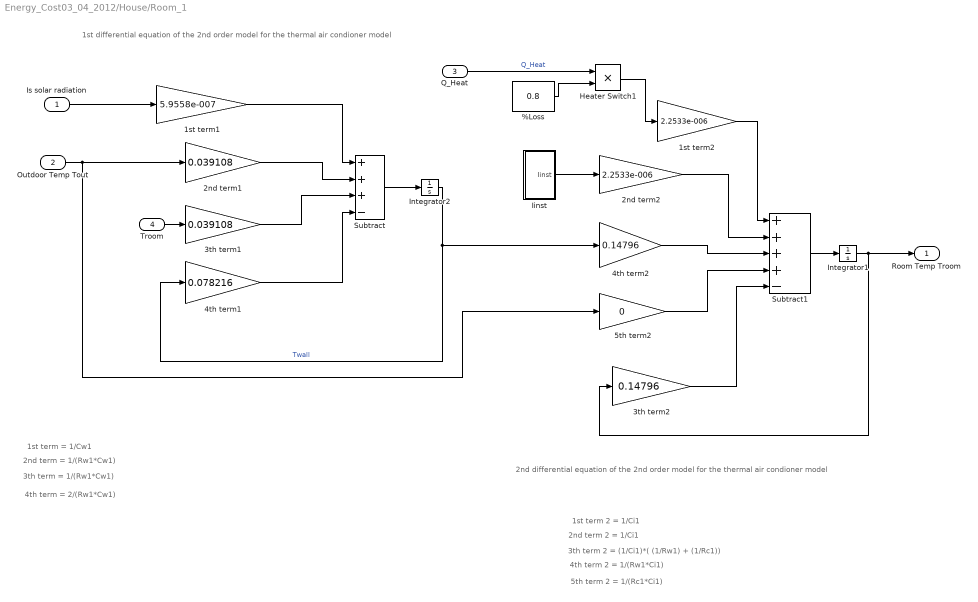
== system Energy_Cost03_04_2012/House/Room_1 ==
  note: 1st differential equation of the 2nd order
      | model for the thermal air condioner model
  note: 2nd differential equation of the 2nd order
      | model for the thermal air condioner model
  note: 1st term = 1/Cw1
  note: 2nd term = 1/(Rw1*Cw1)
  note: 3th term = 1/(Rw1*Cw1)
  note: 4th term = 2/(Rw1*Cw1)
  note: 1st term 2 = 1/Ci1
  note: 2nd term 2 = 1/Ci1
  note: 3th term 2 = (1/Ci1)*( (1/Rw1) + (1/Rc1))
  note: 4th term 2 = 1/(Rw1*Ci1)
  note: 5th term 2 = 1/(Rc1*Ci1)
  Is solar radiation : Inport
  Outdoor Temp Tout : Inport  Port=2
  Q_Heat : Inport  Port=3
  Troom : Inport  Port=4
  %Loss : Constant  Value=0.8
  1st term1 : Gain  Gain=5.9558e-007
  1st term2 : Gain  Gain=2.2533e-006
  2nd term1 : Gain  Gain=0.039108
  2nd term2 : Gain  Gain=2.2533e-006
  3th term1 : Gain  Gain=0.039108
  3th term2 : Gain  Gain=0.14796
  4th term1 : Gain  Gain=0.078216
  4th term2 : Gain  Gain=0.14796
  5th term2 : Gain  Gain=0
  Heater Switch1 : Product  RndMeth=Zero
  Iinst : Subsystem
  Integrator1 : Integrator  InitialCondition=21
  Integrator2 : Integrator  InitialCondition=21
  Subtract : Sum  Inputs=+++-
  Subtract1 : Sum  Inputs=++++-
  Room Temp Troom : Outport  InitialOutput=0
  wires:
  2nd term1/1 -> Subtract/2
  4th term1/1 -> Subtract/4
  Subtract/1 -> Integrator2/1
  Integrator2/1 -> 4th term1/1, 4th term2/1  "Twall"
  Integrator1/1 -> 3th term2/1, Room Temp Troom/1
  Subtract1/1 -> Integrator1/1
  Outdoor Temp Tout/1 -> 2nd term1/1, 5th term2/1
  Troom/1 -> 3th term1/1
  3th term1/1 -> Subtract/3
  1st term1/1 -> Subtract/1
  2nd term2/1 -> Subtract1/2
  Iinst/1(Iinst) -> 2nd term2/1
  Is solar radiation/1 -> 1st term1/1
  4th term2/1 -> Subtract1/3
  5th term2/1 -> Subtract1/4
  3th term2/1 -> Subtract1/5
  Q_Heat/1 -> Heater Switch1/1  "Q_Heat"
  %Loss/1 -> Heater Switch1/2
  1st term2/1 -> Subtract1/1
  Heater Switch1/1 -> 1st term2/1

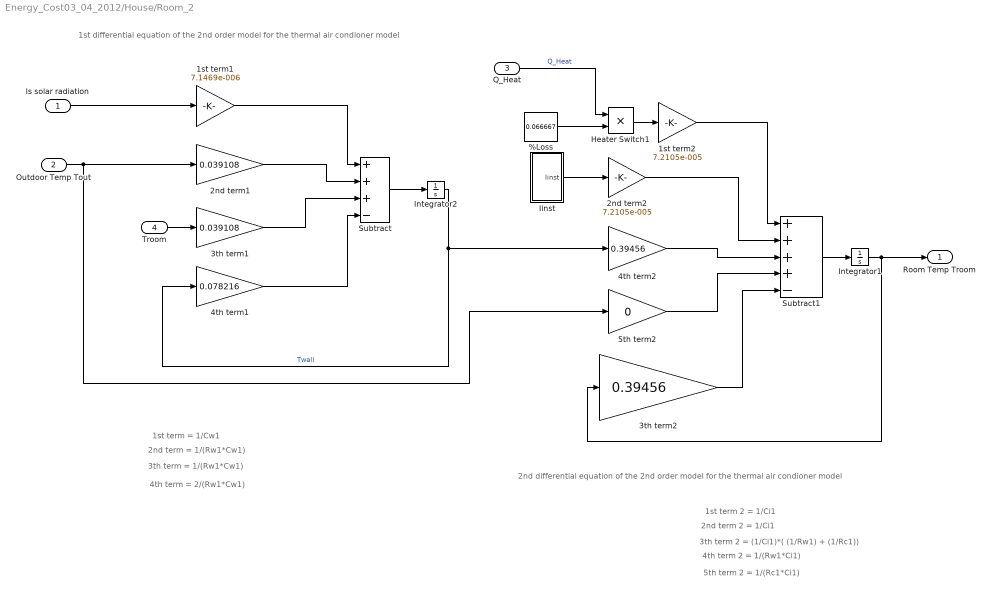
== system Energy_Cost03_04_2012/House/Room_2 ==
  note: 1st differential equation of the 2nd order
      | model for the thermal air condioner model
  note: 2nd differential equation of the 2nd order
      | model for the thermal air condioner model
  note: 1st term = 1/Cw1
  note: 2nd term = 1/(Rw1*Cw1)
  note: 3th term = 1/(Rw1*Cw1)
  note: 4th term = 2/(Rw1*Cw1)
  note: 1st term 2 = 1/Ci1
  note: 2nd term 2 = 1/Ci1
  note: 3th term 2 = (1/Ci1)*( (1/Rw1) + (1/Rc1))
  note: 4th term 2 = 1/(Rw1*Ci1)
  note: 5th term 2 = 1/(Rc1*Ci1)
  Is solar radiation : Inport
  Outdoor Temp Tout : Inport  Port=2
  Q_Heat : Inport  Port=3
  Troom : Inport  Port=4
  %Loss : Constant  Value=0.066667
  1st term1 : Gain  Gain=7.1469e-006
  1st term2 : Gain  Gain=7.2105e-005
  2nd term1 : Gain  Gain=0.039108
  2nd term2 : Gain  Gain=7.2105e-005
  3th term1 : Gain  Gain=0.039108
  3th term2 : Gain  Gain=0.39456
  4th term1 : Gain  Gain=0.078216
  4th term2 : Gain  Gain=0.39456
  5th term2 : Gain  Gain=0
  Heater Switch1 : Product  RndMeth=Zero
  Iinst : Subsystem
  Integrator1 : Integrator  InitialCondition=21
  Integrator2 : Integrator  InitialCondition=21
  Subtract : Sum  Inputs=+++-
  Subtract1 : Sum  Inputs=++++-
  Room Temp Troom : Outport  InitialOutput=0
  wires:
  2nd term1/1 -> Subtract/2
  4th term1/1 -> Subtract/4
  Subtract/1 -> Integrator2/1
  Integrator2/1 -> 4th term1/1, 4th term2/1  "Twall"
  Integrator1/1 -> 3th term2/1, Room Temp Troom/1
  Subtract1/1 -> Integrator1/1
  Outdoor Temp Tout/1 -> 2nd term1/1, 5th term2/1
  Troom/1 -> 3th term1/1
  3th term1/1 -> Subtract/3
  1st term1/1 -> Subtract/1
  2nd term2/1 -> Subtract1/2
  Q_Heat/1 -> Heater Switch1/1  "Q_Heat"
  Iinst/1(Iinst) -> 2nd term2/1
  Is solar radiation/1 -> 1st term1/1
  4th term2/1 -> Subtract1/3
  5th term2/1 -> Subtract1/4
  3th term2/1 -> Subtract1/5
  %Loss/1 -> Heater Switch1/2
  Heater Switch1/1 -> 1st term2/1
  1st term2/1 -> Subtract1/1
